simulink model "probaam"  (R2015a)
settings: Solver=ode45  StartTime=0.0  StopTime=10.0  RelTol=1e-3
settings Model: Creator=Bojana Vasic  LastModifiedBy=Bojana Vasic

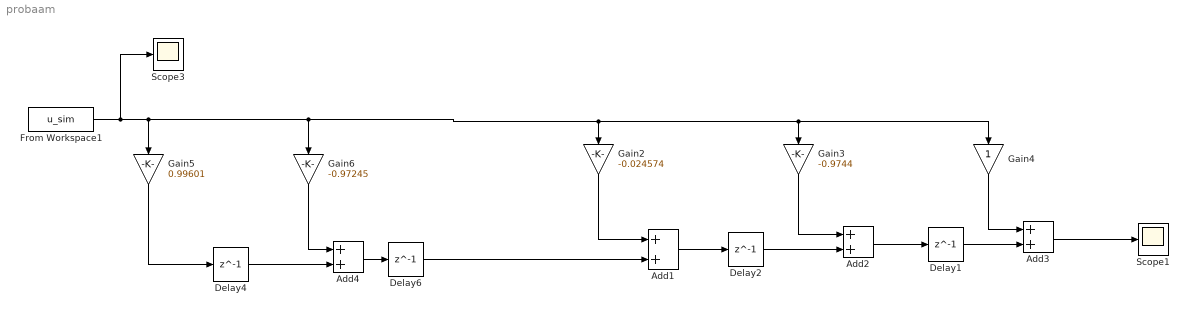
== system probaam ==
  Add{1..4} (4 alike) : Sum
  Delay{1..2,4,6} (4 alike) : Delay  DelayLength=1
  From Workspace1 : FromWorkspace  VariableName=u_sim  SampleTime=1
  Gain2 : Gain  Gain=-0.024574
  Gain3 : Gain  Gain=-0.9744
  Gain4 : Gain
  Gain5 : Gain  Gain=0.99601
  Gain6 : Gain  Gain=-0.97245
  Scope1 : Scope
  Scope3 : Scope
      settings: SaveName=ScopeData3
  wires:
  Gain5/1 -> Delay4/1
  Delay4/1 -> Add4/2
  Gain6/1 -> Add4/1
  Add4/1 -> Delay6/1
  From Workspace1/1 -> Scope3/1, Gain5/1, Gain4/1, Gain3/1, Gain2/1, Gain6/1
  Gain4/1 -> Add3/1
  Gain2/1 -> Add1/1
  Add1/1 -> Delay2/1
  Gain3/1 -> Add2/1
  Delay2/1 -> Add2/2
  Add2/1 -> Delay1/1
  Delay1/1 -> Add3/2
  Add3/1 -> Scope1/1
  Delay6/1 -> Add1/2
